simulink model "testEMplanner_cs"  (R2020b)
settings: Solver=FixedStepAuto  StartTime=0.0  StopTime=inf  FixedStep=1/1000  RelTol=1e-3
PreLoadFcn:
  | mbxruntime.callbacks.PreLoadFcn(bdroot);
PostLoadFcn:
  | mbxruntime.callbacks.PostLoadFcn(bdroot);
InitFcn:
  | mbxruntime.callbacks.InitFcn(bdroot);
StartFcn:
  | mbxruntime.callbacks.StartFcn(bdroot);
StopFcn:
  | mbxruntime.callbacks.StopFcn(bdroot);
model workspace: external: MAT-File testEMplanner_cs_hws.mat (data not in the file)
undefined symbols (not defined in the file): aubr, c_factor, cf, cr, DiscIntNeverNeededParam, global_path_x, global_path_y, KD_PID_distance, KD_PID_speed, KI_PID_distance, KI_PID_speed, KP_PID_distance, KP_PID_speed, la, lb, LQR_K1, LQR_K2, LQR_K3, LQR_K4, m, rack_displacement, right_wheel_ground, tablebr, vubr, vx_break_point
libraries: PreScanSimulinkLibrary x38, Solver_SF x1
(part 12 of 16)

== matlab function testEMplanner_cs/Audi_A8_Sedan_1/decision&planning module with quad1/EM Planner/obs/MATLAB Function2 ==
  data: x_set input; match_point_index_set output; y_set input; frenet_path_x input; frenet_path_y input; frenet_path_heading input; frenet_path_kappa input; proj_x_set output; proj_y_set output; proj_heading_set output; proj_kappa_set output
function [match_point_index_set,proj_x_set, proj_y_set,proj_heading_set,proj_kappa_set] = ...
    fcn(x_set,y_set,frenet_path_x,frenet_path_y,frenet_path_heading,frenet_path_kappa)
%该函数将批量计算x_set，y_set中的xy，在frenet_path下的投影的信息
%输入 x_set,y_set，待投影的点的集合
%x_set,y_set,frenet_path_x,frenet_path_y,frenet_path_heading,frenet_path_kappa
%曲线在直角坐标系下的x，y，heading，kappa
%输出：match_point_index_set 匹配点在frenet_path下的编号的集合(即从全局路径第一个点开始数，第几个点是匹配点)
%     proj_x y heading kappa 投影的x,y,heading,kappa的集合

% 由于事先不知道x_set中到底有多少个点需要投影，因此事先声明一个最大的数量的点作为缓冲
n = 128;
% 并且由于不知道投影点的个数，所以也不知道输出的个数，因此输出也要做缓冲，用nan表示不存在的点
% 输出最多输出128个
% 输出初始化
match_point_index_set = ones(n,1) * nan;
proj_x_set = ones(n,1) * nan;
proj_y_set = ones(n,1) * nan;
proj_heading_set = ones(n,1) * nan;
proj_kappa_set = ones(n,1) * nan;

% 找匹配点，需要利用上一个周期的结果作为下一个周期遍历的起点，因此需要声明两个全局变量

persistent is_first_run;
persistent pre_match_point_index_set;%bug :pre_match_point_index(i) 未必代表的是第i个障碍物的match_point_index
persistent pre_frenet_path_x;
persistent pre_frenet_path_y;
persistent pre_frenet_path_heading;
persistent pre_frenet_path_kappa;
persistent pre_x_set;
persistent pre_y_set;
%算法主函数入口

if isempty(is_first_run)
    %该if分支表示函数首次运行
    is_first_run = 0;
    pre_frenet_path_x = frenet_path_x;
    pre_frenet_path_y = frenet_path_y;
    pre_frenet_path_heading = frenet_path_heading;
    pre_frenet_path_kappa = frenet_path_kappa;
    %要记录首次运行计算的匹配点的结果供下个周期运行，先初始化
    pre_match_point_index_set = ones(n,1) * nan;
    %对x_set,y_set的点做遍历，找到他们的匹配点
    for i = 1 : length(x_set)
        if isnan(x_set(i))
            break;
        end
        %首次运行时，没有任何提示，只能从frenet path的第一个点开始找
        start_search_index = 1;
        % 声明increase_count，用于表示在遍历时distance连续增加的个数
        increase_count = 0;
        % 开始遍历
        min_distance = inf;
        for j = start_search_index : length(frenet_path_x)
            distance = (x_set(i) - frenet_path_x(j))^2 + (y_set(i) - frenet_path_y(j))^2;
            if distance < min_distance
                min_distance = distance;
                match_point_index_set(i) = j;
                increase_count = 0;
            else
                increase_count = increase_count + 1;
            end
            %如果distance连续增加50次就不要再遍历了，节省时间
            if increase_count > 50
                break;
            end
        end
        
        %如何通过匹配点计算投影点，请参见《自动驾驶控制算法第七讲》
        %或《自动驾驶决策规划算法》第一章第三节
        
        %取出匹配点的编号
        match_point_index = match_point_index_set(i);
        %取出匹配点的信息
        match_point_x = frenet_path_x(match_point_index);
        match_point_y = frenet_path_y(match_point_index);
        match_point_heading = frenet_path_heading(match_point_index);
        match_point_kappa = frenet_path_kappa(match_point_index);
        %计算匹配点的方向向量与法向量
        vector_match_point = [match_point_x;match_point_y];
        vector_match_point_direction = [cos(match_point_heading);sin(match_point_heading)];
        %声明待投影点的位矢
        vector_r = [x_set(i);y_set(i)];
        
       %通过匹配点计算投影点
       vector_d = vector_r - vector_match_point;
       ds = vector_d' * vector_match_point_direction;
       vector_proj_point = vector_match_point + ds * vector_match_point_direction;
       proj_heading = match_point_heading + match_point_kappa * ds;
       proj_kappa = match_point_kappa;
       %计算结果输出
       proj_x_set(i) = vector_proj_point(1);
       proj_y_set(i) = vector_proj_point(2);
       proj_heading_set(i) = proj_heading;
       proj_kappa_set(i) = proj_kappa;
    end
    %匹配点的计算结果保存，供下一个周期使用
    pre_match_point_index_set = match_point_index_set;
    pre_x_set = x_set;
    pre_y_set = y_set;
else
    %此if分支表示不是首次运行
    %对每个x_set上的点做处理
    for i = 1 : length(x_set)
        %不是首次运行，对于点x_set(i),y_set(i)来说,start_search_index =
        %pre_match_point_index_set(i)
        start_search_index = pre_match_point_index_set(i);%上个周期匹配点的编号作为本周期搜索的起点
        % 判断帧与帧之间的障碍物是否为同一个
        square_dis = (x_set(i) - pre_x_set(i))^2 + (y_set(i) - pre_y_set(i))^2;
        if square_dis > 36
            % 帧与帧之间的物体的位置距离过大，认为是两个障碍物
            start_search_index = nan;
        end
        % 声明increase_count，用于表示在遍历时distance连续增加的个数
        %%%%%%%%%
        %对于障碍物检测而言，当感知第一次检测到障碍物时，算法并不是首次运行，此时 
        %pre_match_point_index_set的值是nan，如果还用上一时刻的结果作为本周期搜索的起点
        %必然会出问题，所以要修改
        % 声明increase_count_limit
        increase_count_limit = 5;
        if isnan(start_search_index)
            %没有上个周期的结果，那就不能只检查5次了
            increase_count_limit = 50;
            %搜索起点也要设为1
            start_search_index = 1;
        end
        increase_count = 0;
        % 开始遍历
        %这里多一个步骤，判断遍历的方向
        %计算上个周期匹配点的位矢
        vector_pre_match_point = [pre_frenet_path_x(start_search_index);pre_frenet_path_y(start_search_index)];
        vector_pre_match_point_direction = ...
            [cos(pre_frenet_path_heading(start_search_index));sin(pre_frenet_path_heading(start_search_index))];
        %判断遍历的方向
        flag = ([x_set(i);y_set(i)] - vector_pre_match_point)' * vector_pre_match_point_direction;
        min_distance = inf;
        if flag > 0.001
            for j = start_search_index : length(frenet_path_x)
                distance = (x_set(i) - frenet_path_x(j))^2 + (y_set(i) - frenet_path_y(j))^2;
                if distance < min_distance
                    min_distance = distance;
                    match_point_index_set(i) = j;
                    increase_count = 0;
                else
                    increase_count = increase_count + 1;
                end
                %如果distance连续增加increase_count_limit次就不要再遍历了，节省时间
                if increase_count > increase_count_limit
                    break;
                end
            end
        elseif flag < - 0.001
            for j = start_search_index : -1 : 1
                distance = (x_set(i) - frenet_path_x(j))^2 + (y_set(i) - frenet_path_y(j))^2;
                if distance < min_distance
                    min_distance = distance;
                    match_point_index_set(i) = j;
                    increase_count = 0;
                else
                    increase_count = increase_count + 1;
                end
                %如果distance连续增加increase_count_limit次就不要再遍历了，节省时间
                if increase_count > increase_count_limit
                    break;
                end
            end
        else
            match_point_index_set(i) = start_search_index;
        end
        
        %如何通过匹配点计算投影点，请参见《自动驾驶控制算法第七讲》
        %或《自动驾驶决策规划算法》第一章第三节
        
        %取出匹配点的编号
        match_point_index = match_point_index_set(i);
        %取出匹配点的信息
        match_point_x = frenet_path_x(match_point_index);
        match_point_y = frenet_path_y(match_point_index);
        match_point_heading = frenet_path_heading(match_point_index);
        match_point_kappa = frenet_path_kappa(match_point_index);
        %计算匹配点的方向向量与法向量
        vector_match_point = [match_point_x;match_point_y];
        vector_match_point_direction = [cos(match_point_heading);sin(match_point_heading)];
        %声明待投影点的位矢
        vector_r = [x_set(i);y_set(i)];
        
       %通过匹配点计算投影点
       vector_d = vector_r - vector_match_point;
       ds = vector_d' * vector_match_point_direction;
       vector_proj_point = vector_match_point + ds * vector_match_point_direction;
       proj_heading = match_point_heading + match_point_kappa * ds;
       proj_kappa = match_point_kappa;
       %计算结果输出
       proj_x_set(i) = vector_proj_point(1);
       proj_y_set(i) = vector_proj_point(2);
       proj_heading_set(i) = proj_heading;
       proj_kappa_set(i) = proj_kappa;
  
    end
    %匹配点的计算结果保存，供下一个周期使用
    pre_match_point_index_set = match_point_index_set;
    pre_frenet_path_x = frenet_path_x;
    pre_frenet_path_y = frenet_path_y;
    pre_frenet_path_heading = frenet_path_heading;
    pre_frenet_path_kappa = frenet_path_kappa;
    pre_x_set = x_set;
    pre_y_set = y_set;
end

== matlab function testEMplanner_cs/Audi_A8_Sedan_1/decision&planning module with quad1/EM Planner/obs/obs filter ==
  data: host_x input; obs_x_set_final output; host_y input; host_heading_xy input; obs_x_set_gcs input; obs_y_set_gcs input; obs_velocity_set_gcs input; obs_heading_set_gcs input; obs_y_set_final output; obs_velocity_set_final output; obs_heading_set_final output
function [obs_x_set_final,obs_y_set_final,obs_velocity_set_final,obs_heading_set_final] = fcn(host_x,host_y,host_heading_xy,obs_x_set_gcs,obs_y_set_gcs,obs_velocity_set_gcs,obs_heading_set_gcs)
% 该函数将筛选障碍物，纵向[-10,60] 横向[-10,10]的障碍物才会被考虑
% 该函数只是一种单车道的临时办法，考虑到多车道情况，即使障碍物距离较远也应该考虑
% EM Planner完全体是多车道并行计算的，每个车道都生成参考线然后并行计算出多条轨迹，再选择最优的轨迹作为输出

%传感器最多可以识别32个障碍物
n = 32;
%输出初始化
obs_x_set_final = ones(n,1)*nan;
obs_y_set_final = ones(n,1)*nan;
obs_velocity_set_final = ones(n,1)*nan;
obs_heading_set_final = ones(n,1)*nan;
count = 1;
for i = 1:length(obs_x_set_gcs)
    if isnan(obs_x_set_gcs(i))
        break;
    end
    %自车的heading的方向向量与法向量
    tor = [cos(host_heading_xy);sin(host_heading_xy)];
    nor = [-sin(host_heading_xy);cos(host_heading_xy)];
    %障碍物与自车的距离向量
    vector_obs = [obs_x_set_gcs(i);obs_y_set_gcs(i)] - [host_x;host_y];
    %障碍物纵向距离
    lon_distance = vector_obs'*tor;
    %障碍物横向距离
    lat_distance = vector_obs'*nor;
    
    if (lon_distance < 60) && (lon_distance > -10) && (lat_distance > -10) && (lat_distance < 10)
        obs_x_set_final(count) = obs_x_set_gcs(i);
        obs_y_set_final(count) = obs_y_set_gcs(i);
        obs_heading_set_final(count) = obs_heading_set_gcs(i);
        obs_velocity_set_final(count) = obs_velocity_set_gcs(i);
        count = count + 1;
    end
end

== matlab function testEMplanner_cs/Audi_A8_Sedan_1/decision&planning module with quad1/EM Planner/path and speed merge ==
  data: s input; trajectory_x output; s_dot input; s_dot2 input; relative_time input; current_time input; path_s input; trajectory_x_init input; trajectory_y_init input; trajectory_heading_init input; trajectory_kappa_init input; trajectory_y output; trajectory_heading output; trajectory_kappa output; trajectory_speed output; trajectory_accel output; trajectory_time output
function [trajectory_x,trajectory_y,trajectory_heading,trajectory_kappa,trajectory_speed,trajectory_accel,trajectory_time] = ...
    fcn(s,s_dot,s_dot2,relative_time,current_time,path_s,trajectory_x_init,trajectory_y_init,trajectory_heading_init,trajectory_kappa_init)
% 该函数将合并path和speed
% 由于path 是 60个点，speed 有 401个点，合并后，path和speed有401个点，因此需要做插值
n = 401;
trajectory_x = zeros(n,1);
trajectory_y = zeros(n,1);
trajectory_heading = zeros(n,1);
trajectory_kappa = zeros(n,1);
trajectory_speed = zeros(n,1);

trajectory_accel = zeros(n,1);
index = 1;
% 由于trajectory_x_init中不是所有的值都有效，(有nan) 所以要找到有效值的范围
while ~isnan(trajectory_x_init(index)) 
    index = index + 1;
end
index = index - 1;
trajectory_time = zeros(n,1);
for i = 1:n-1
    %interp1 线性插值
    % 若 x = [1,2] y = [3,4]
    %interp1(x,y,1.5) 会得到3.5
    %interp1 的缺点是 在端点或超过端点的，结果为nan
    % interp1(x,y,2) 不会等于4 而是会等于nan
    % interp1(x,y,6) 也会等于nan，所以在端点处要单独处理
    trajectory_x(i) = interp1(path_s(1:index),trajectory_x_init(1:index),s(i));
    trajectory_y(i) = interp1(path_s(1:index),trajectory_y_init(1:index),s(i));
    trajectory_heading(i) = interp1(path_s(1:index),trajectory_heading_init(1:index),s(i));
    trajectory_kappa(i) = interp1(path_s(1:index),trajectory_kappa_init(1:index),s(i));
    trajectory_time(i) = relative_time(i) + current_time;%速度规划会得到相对时间，转换成绝对时间
    trajectory_speed(i) = s_dot(i);
    trajectory_accel(i) = s_dot2(i);
end
% 端点单独处理
trajectory_x(end) = trajectory_x_init(end);
trajectory_y(end) = trajectory_y_init(end);
trajectory_heading(end) = trajectory_heading_init(end);
trajectory_kappa(end) = trajectory_kappa_init(end);
trajectory_time(end) = relative_time(end) + current_time;
trajectory_speed(end) = s_dot(end);
trajectory_accel(end) = s_dot2(end);

== matlab function testEMplanner_cs/Audi_A8_Sedan_1/decision&planning module with quad1/EM Planner/path decision task/increase DP path nodes ==
  data: dp_path_s_init input; dp_path_s_final output; dp_path_l_init input; plan_start_s input; plan_start_l input; plan_start_dl input; plan_start_ddl input; dp_path_l_final output; dp_path_dl_final output; dp_path_ddl_final output
function [dp_path_s_final,dp_path_l_final,dp_path_dl_final,dp_path_ddl_final] = ...
    fcn(dp_path_s_init,dp_path_l_init,plan_start_s,plan_start_l,plan_start_dl,plan_start_ddl)
% 该函数将增密dp_path_s,dp_path_l
% 由于事先不知道动态规划采样的行和列，也就不知道动态规划计算的曲线有多长，因此需要做缓冲
% 每1“米”采样一个点，一共采60个
ds = 1;
% 输出初始化
dp_path_s_final = ones(60,1)*nan;
dp_path_l_final = ones(60,1)*nan;
dp_path_dl_final = ones(60,1)*nan;
dp_path_ddl_final = ones(60,1)*nan;

% 设置五次多项式的起点
start_s = plan_start_s;
start_l = plan_start_l;
start_dl = plan_start_dl;
start_ddl = plan_start_ddl;

s_cur = [];
l_temp = [];
dl_temp =[];
ddl_temp = [];

for i = 1:length(dp_path_s_init)
    if dp_path_s_init(i) == -1
        break;
    end
    for j = 1:10000
        %采样s
        s_node = start_s + ds*(j - 1);
        if s_node < dp_path_s_init(i)
            s_cur = [s_cur,s_node];
        else
            break;
        end
    end
    end_s = dp_path_s_init(i);
    end_l = dp_path_l_init(i);
    end_dl = 0;
    end_ddl = 0;
    coeff = CalcQuinticCoeffient(start_l,start_dl,start_ddl,end_l,end_dl,end_ddl,start_s,end_s);
    a0 = coeff(1);
    a1 = coeff(2);
    a2 = coeff(3);
    a3 = coeff(4);
    a4 = coeff(5);
    a5 = coeff(6);
    l = a0 * ones(1,length(s_cur)) + a1 * s_cur + a2 * s_cur.^2 + a3 * s_cur.^3 +...
        a4 * s_cur.^4 + a5 * s_cur.^5;
    dl = a1 * ones(1,length(s_cur)) + 2 * a2 * s_cur + 3 * a3 * s_cur.^2 + ...
        4 * a4 * s_cur.^3 + 5 * a5 * s_cur.^4;
    ddl = 2 * a2 * ones(1,length(s_cur)) + 6 * a3 * s_cur + 12 * a4 * s_cur.^2 + ...
        20 * a5 * s_cur.^3;
    % 把 l dl ddl 的结果保存
    l_temp = [l_temp,l];
    dl_temp = [dl_temp,dl];
    ddl_temp = [ddl_temp,ddl];
    % end的值赋值给start 做下一步循环
    start_s = end_s;
    start_l = end_l;
    start_dl = end_dl;
    start_ddl = end_ddl;
    s_cur = [];
end
   for k = 1:length(l_temp)
       if k == 61
           break;
       end
       dp_path_s_final(k) = plan_start_s + ds * (k - 1);
       dp_path_l_final(k) = l_temp(k);
       dp_path_dl_final(k) = dl_temp(k);
       dp_path_ddl_final(k) = ddl_temp(k);
   end
end

function coeff = CalcQuinticCoeffient(start_l,start_dl,start_ddl,end_l,end_dl,end_ddl,start_s,end_s)
    % l = a0 + a1*s + a2*s^2 + a3*s^3 + a4*s^4 + a5*s^5
    % l' = a1 + 2 * a2 * s + 3 * a3 * s^2 + 4 * a4 * s^3 + 5 * a5 * s^4
    % l'' = 2 * a2 + 6 * a3 * s + 12 * a4 * s^2 + 20 * a5 * s^3
    start_s2 = start_s * start_s;
    start_s3 = start_s2 * start_s;
    start_s4 = start_s3 * start_s;
    start_s5 = start_s4 * start_s;
    end_s2 = end_s * end_s;
    end_s3 = end_s2 * end_s;
    end_s4 = end_s3 * end_s;
    end_s5 = end_s4 * end_s;
    A = [1,start_s, start_s2,     start_s3,     start_s4,      start_s5;
         0 1,       2 * start_s,  3 * start_s2, 4 * start_s3,  5 * start_s4;
         0 0,       2,            6 * start_s,  12 * start_s2, 20 * start_s3;
         1,end_s, end_s2,     end_s3,     end_s4,      end_s5;
         0,1,     2 * end_s,  3 * end_s2, 4 * end_s3,  5 * end_s4;
         0,0,     2,          6 * end_s,  12 * end_s2, 20 * end_s3;];
    B = [start_l;
         start_dl;
         start_ddl;
         end_l;
         end_dl;
         end_ddl;];
     coeff = A \ B;
    
end

== matlab function testEMplanner_cs/Audi_A8_Sedan_1/decision&planning module V0.1/EM Planner/calc plan start info and stitch trajectory ==
  data: pre_trajectory_x input; plan_start_x output; pre_trajectory_y input; pre_trajectory_heading input; pre_trajectory_kappa input; pre_trajectory_velocity input; pre_trajectory_accel input; pre_trajectory_time input; current_time input; host_x input; host_y input; host_heading_xy input; host_vx input; host_vy input; host_ax input; host_ay input; plan_start_y output; plan_start_heading output; plan_start_kappa output; plan_start_vx output; plan_start_vy output; plan_start_ax output; plan_start_ay output; plan_start_time output; stitch_x output; stitch_y output; stitch_heading output; stitch_kappa output; stitch_speed output; stitch_accel output; stitch_time output
function [plan_start_x,plan_start_y,plan_start_heading,plan_start_kappa,plan_start_vx,plan_start_vy,plan_start_ax,...
    plan_start_ay,plan_start_time,stitch_x,stitch_y,stitch_heading,stitch_kappa,stitch_speed,stitch_accel,stitch_time] ...
    = fcn(pre_trajectory_x,pre_trajectory_y,pre_trajectory_heading,pre_trajectory_kappa,pre_trajectory_velocity,...
    pre_trajectory_accel,pre_trajectory_time,current_time,host_x,host_y,host_heading_xy,host_vx,host_vy,host_ax,host_ay)
%该函数将计算规划的起点以及拼接轨迹的信息
%输入 上一周期的规划结果信息pre_trajectory x ,y,heading,kappa,velocity,accel,time
%     本周期的绝对时间current_time
%     定位信息host x,y,heading,kappa,vx,vy,ax,ay
%输出 规划起点信息plan_start x,y,heading,kappa,vx,vy,ax,ay(vx,vy,ax,ay)是世界坐标系的
%     待拼接的轨迹信息，一般在上一周期的轨迹中的current_time+100ms，往前取20个点。
%     当规划完成后，本周期的规划结果和stitch_trajectory一起拼好发给控制

%输出初始化
stitch_x = zeros(20,1);
stitch_y = zeros(20,1);
stitch_heading = zeros(20,1);
stitch_kappa = zeros(20,1);
stitch_speed = zeros(20,1);
stitch_accel = zeros(20,1);
%时间为负代表没有对应的拼接轨迹
stitch_time = ones(20,1)*-1;

%申明全局变量
persistent is_first_run;
if isempty(is_first_run)
    %代表代码首次运行
    is_first_run = 0;
    %按照轨迹拼接算法，应该用车辆动力学递推，但是首次运行车辆的速度都是0，所以没必要递推了
    plan_start_x = host_x;
    plan_start_y = host_y;
    plan_start_heading = host_heading_xy;
    plan_start_kappa = 0;
    plan_start_vx = 0;
    plan_start_vy = 0;
    plan_start_ax = 0;
    plan_start_ay = 0;
    %规划的起点的时间应该是当前时间+100ms
    plan_start_time = current_time + 0.1;
else
    %该函数不是首次运行
    x_cur = host_x;
    y_cur = host_y;
    heading_cur = host_heading_xy;
    kappa_cur = 0;
    %vx vy ax ay要转换成世界坐标系
    vx_cur = host_vx*cos(heading_cur) - host_vy*sin(heading_cur);
    vy_cur = host_vx*sin(heading_cur) + host_vy*cos(heading_cur);
    ax_cur = host_ax*cos(heading_cur) - host_ay*sin(heading_cur);
    ay_cur = host_ax*sin(heading_cur) + host_ay*cos(heading_cur);
    %规划周期
    dt = 0.1;
    %由于不是首次运行了，有上一时刻的轨迹了，找到上一周期轨迹规划的本周期车辆应该在的位置
    for i = 1:length(pre_trajectory_time) - 1
        if (pre_trajectory_time(i) <= current_time && pre_trajectory_time(i + 1) > current_time)
            break;
        end
    end
    %上一周期规划的本周期的车应该在的位置
    pre_x_desire = pre_trajectory_x(i);
    pre_y_desire = pre_trajectory_y(i);
    pre_heading_desire = pre_trajectory_heading(i);
    %计算横纵向误差
    %切向量
    tor = [cos(pre_heading_desire);sin(pre_heading_desire)];
    %法向量
    nor = [-sin(pre_heading_desire);cos(pre_heading_desire)];
    %误差向量
    d_err = [host_x;host_y] - [pre_x_desire;pre_y_desire];
    %纵向误差
    lon_err = abs(d_err'*tor);
    %横向误差
    lat_err = abs(d_err'*nor);
    %纵向误差大于2.5 横向误差大于0.5 认为控制没跟上
    if (lon_err > 2.5)||(lat_err > 0.5)
        %此分支处理控制未跟上的情况，规划起点通过运动学递推
        plan_start_x = x_cur + vx_cur * dt + 0.5 * ax_cur * dt * dt;
        plan_start_y = y_cur + vy_cur * dt + 0.5 * ay_cur * dt * dt;
        plan_start_vx = vx_cur + ax_cur * dt;
        plan_start_vy = vy_cur + ay_cur * dt;
        plan_start_heading = atan2(plan_start_vy,plan_start_vx);
        plan_start_ax = ax_cur;
        plan_start_ay = ay_cur;
        plan_start_kappa = kappa_cur;
        plan_start_time = current_time + 0.1;
        return;
    else
        %此分支表示控制能跟的上规划，开始拼接
        for j = i:length(pre_trajectory_time) - 1
            if (pre_trajectory_time(j) <= current_time + 0.1)&&(pre_trajectory_time(j + 1) > current_time + 0.1)
                break;
            end
        end
        %注：此算法要能运行需要trajectory的点有很高的密度
        plan_start_x = pre_trajectory_x(j);
        plan_start_y = pre_trajectory_y(j);
        plan_start_heading = pre_trajectory_heading(j);
        plan_start_kappa = pre_trajectory_kappa(j);
        %这里的pre_trajectory的速度,加速度是指轨迹的切向速度，切向加速度
        plan_start_vx = pre_trajectory_velocity(j) * cos(plan_start_heading);
        plan_start_vy = pre_trajectory_velocity(j) * sin(plan_start_heading);
        %pre_trajectory的加速度是切向加速度，要想计算ax,ay还要计算法向加速度
        %计算轨迹在current_time + 100ms 这个点的切向量法向量
        tor = [cos(plan_start_heading);sin(plan_start_heading)];
        nor = [-sin(plan_start_heading);cos(plan_start_heading)];
        a_tor = pre_trajectory_accel(j) * tor;
        a_nor = pre_trajectory_velocity(j)^2 * plan_start_kappa * nor ;
        plan_start_ax = a_tor(1) + a_nor(1);
        plan_start_ay = a_tor(2) + a_nor(2);
        plan_start_time = pre_trajectory_time(j);
        %计算拼接轨迹
        %j 表示 current_time + 0.1 的时间点在 pre_trajectory_time的编号
        %拼接是往从j开始，往前拼接20个，也就是pre_trajectory(j-1),j-2,j-3,....j-19
        %分两种情况，如果j小于20，意味着前面的轨迹点不够20个
        %如果j >= 20,意味着前面的点多于20个
        %还有一个细节需要考虑，pre_trajectory x(j) y(j) ....是规划的起点，那么在轨迹拼接时
        %需不需要在stitch_trajectory中把pre_trajectory x(j) y(j) ....包含进去
        %答案是否定的，不应该包进去，因为规划的起点会在规划模块计算完成后的结果中包含，如果在拼接的时候
        %还要包含，那就等于规划起点包含了两次
        %除非本周期计算的轨迹不包含规划起点，那么stitch_trajectory可以包含规划起点。
        %如果本周期计算的轨迹包含规划起点，那么stitch_trajectory就不可以包含规划起点。
        %我们选择规划包含起点，拼接不包含起点的做法
        
        %把起点去掉
        j = j - 1;
        if j >= 20
            stitch_x = pre_trajectory_x(j - 19:j);
            stitch_y = pre_trajectory_y(j - 19:j);
            stitch_heading = pre_trajectory_heading(j - 19:j);
            stitch_kappa = pre_trajectory_kappa(j - 19:j);
            stitch_speed = pre_trajectory_velocity(j - 19:j);
            stitch_accel = pre_trajectory_accel(j - 19:j);
            stitch_time = pre_trajectory_time(j - 19:j);
        else
            stitch_x(20 - j + 1:20) = pre_trajectory_x(1:j);
            stitch_y(20 - j + 1:20) = pre_trajectory_y(1:j);
            stitch_heading(20 - j + 1:20) = pre_trajectory_heading(1:j);
            stitch_kappa(20 - j + 1:20) = pre_trajectory_kappa(1:j);
            stitch_speed(20 - j + 1:20) = pre_trajectory_velocity(1:j);
            stitch_accel(20 - j + 1:20) = pre_trajectory_accel(1:j);
            stitch_time(20 - j + 1:20) = pre_trajectory_time(1:j);           
        end   
    end    
end

== matlab function testEMplanner_cs/Audi_A8_Sedan_1/decision&planning module with quad1/EM Planner/path decision task/path decision with dynamic planning(dp) ==
  data: obs_s_set input; dp_path_s output; obs_l_set input; plan_start_s input; plan_start_l input; plan_start_dl input; plan_start_dll input; w_cost_collision input; w_cost_smooth_dl input; w_cost_smooth_ddl input; w_cost_smooth_dddl input; w_cost_ref input; row input; col input; sample_s input; sample_l input; dp_path_l output
function [dp_path_s,dp_path_l] = fcn(obs_s_set,obs_l_set,plan_start_s,plan_start_l,plan_start_dl,...
    plan_start_dll,w_cost_collision,w_cost_smooth_dl,w_cost_smooth_ddl,w_cost_smooth_dddl,w_cost_ref,row,col,sample_s,sample_l)
%该函数为路径决策算法动态规划的主函数
% 输入：obs s l set 筛选后的障碍物sl信息
%       plan_start s l dl ddl 规划起点信息
%       w_cost_obs,w_cost_smooth_dl,w_cost_smooth_ddl,w_cost_smooth_dddl,w_cost_ref动态规划代价权重
%       row col 动态规划采样点的行数和列数(row必须是奇数，col必须是6)
%       sample_s,sample_l 采样的s l 长度
% 输出：dp_path_l,dp_path_s 动态规划的路径sl,此路径不包含规划起点  

%动态规划最优的数据结构是结构体矩阵，但是simulink不支持结构体矩阵，所以动态规划算法写的相对难以理解

%声明二维矩阵变量node_cost，node_cost(i,j)表示从起点出发，到行i列j节点的最小代价为node_cost(i,j)
node_cost = ones(row,col)*inf;%初始化为无穷大

%声明二维矩阵变量pre_node_index pre_node_index(i,j)表示从起点到行i列j的节点的最优路径中前一个节点的行号为
%pre_node_index(i,j)
%例：比如一条最优路径为 起点 -> node(1,1) -> node(2,2) -> node(3,3)
%则pre_node_index(3,3) = 2 (最优路径的前一个节点是node(2,2) 取它的行号）
%  pre_node_index(2,2) = 1 (最优路径的前一个节点是node(1,1) 取它的行号）
%  pre_node_index(1,1) = 0 (起点的行号默认是0)

% 其实pre_node_index就是当找到最小代价的路径后从终点到起点反向选择出最优路径的
%如果用结构体矩阵完全没有必要弄得这么麻烦，但是simulink不支持
pre_node_index = zeros(row,col);%初始化，所有节点的上个最优节点的行号都是0，也就是起点

%先计算从起点到第一列的cost
for i = 1:row
    node_cost(i,1) = CalcStartCost(plan_start_s,plan_start_l,plan_start_dl,...
    plan_start_dll,i,sample_s,sample_l,w_cost_collision,w_cost_smooth_dl,...
    w_cost_smooth_ddl,w_cost_smooth_dddl,w_cost_ref,obs_s_set,obs_l_set,row);
end
% 动态规划主函数，从第二列开始
for j = 2:col
    for i = 1:row
        %计算当前node(i,j)的s l
        cur_node_s = plan_start_s + j * sample_s;
        cur_node_l = ((row + 1)/2 - i) * sample_l;
        %遍历前一列的节点
        for k = 1:row
            %计算前一列节点的s l
            pre_node_s = plan_start_s + (j - 1) * sample_s;
            pre_node_l = ((row + 1)/2 - k) * sample_l;
            cost_neighbour = CalcNeighbourCost(pre_node_s,pre_node_l,cur_node_s,cur_node_l,w_cost_collision,...
    w_cost_smooth_dl,w_cost_smooth_ddl,w_cost_smooth_dddl,w_cost_ref,obs_s_set,obs_l_set);
            %起点到上一个节点的最小代价为node_cost(k,j-1)
            pre_min_cost = node_cost(k,j-1);
            %起点到node_cost(i,j)的最小代价 为node_cost(k,j-1)
            %再加上node(k,j-1)到node(i,j)的代价 (k = 1,2,3,4...row) 中最小的
            cost_temp = pre_min_cost + cost_neighbour;
            if cost_temp < node_cost(i,j)
                node_cost(i,j) = cost_temp;
                %把最优路径上一列节点的行号记录下来
                pre_node_index(i,j) = k;
            end
        end      
    end
end
%找到node_cost最后一列中，cost最小的，记代价最小的行号为index
index = 0;
min_cost = inf;
for i = 1:row
    if node_cost(i,end) < min_cost
        min_cost = node_cost(i,end);
        index = i;
    end
end
%动态规划最优路径初始化
dp_node_list_row = zeros(col,1);
%从后往前逆推
cur_index = index;
for i = 1:col
    %记录cur_index前面节点的行号
    pre_index = pre_node_index(cur_index,end - i + 1);
    %把cur_index放到dp_node_list_row对应的位置
    dp_node_list_row(col - i + 1) = cur_index;
    %再把pre_index 赋给 cur_index 进行下一步递推
    cur_index = pre_index;
end
% 输出初始化，由于事先不知道横纵向的采样列数，因此需要做缓冲
dp_path_s = ones(15,1)*-1;
dp_path_l = ones(15,1)*-1;
for i = 1:col
    dp_path_s(i) = plan_start_s + i * sample_s;
    dp_path_l(i) = ((row + 1) / 2 - dp_node_list_row(i)) * sample_l;
end








end
function cost = CalcNeighbourCost(pre_node_s,pre_node_l,cur_node_s,cur_node_l,w_cost_collision,...
    w_cost_smooth_dl,w_cost_smooth_ddl,w_cost_smooth_dddl,w_cost_ref,obs_s_set,obs_l_set)
% 该函数将计算相邻两个节点之间的cost
  
    start_l = pre_node_l;
    start_dl = 0;
    start_ddl = 0;
    end_l = cur_node_l;
    end_dl = 0;
    end_ddl = 0;
    start_s = pre_node_s;
    end_s = cur_node_s;
    coeff = CalcQuinticCoeffient(start_l,start_dl,start_ddl,end_l,end_dl,end_ddl,start_s,end_s);
    a0 = coeff(1);
    a1 = coeff(2);
    a2 = coeff(3);
    a3 = coeff(4);
    a4 = coeff(5);
    a5 = coeff(6);
    % 取10个点计算cost
    ds = zeros(10,1);
    l = zeros(10,1);
    dl = zeros(10,1);
    ddl = zeros(10,1);
    dddl = zeros(10,1);
    for i = 1:10
        ds(i) = start_s + (i-1)*(end_s - start_s)/10;
    end
    l = a0 * ones(10,1) + a1 * ds + a2 * ds.^2 + a3 * ds.^3 + a4 * ds.^4 + a5 * ds.^5;
    dl = a1 * ones(10,1) + 2 * a2 * ds + 3 * a3 * ds.^2 + 4 * a4 * ds.^3 + 5 * a5 * ds.^4;
    ddl = 2 * a2 * ones(10,1) + 6 * a3 * ds + 12 * a4 * ds.^2 + 20 * a5 * ds.^3;
    dddl = 6 * ones(10,1) * a3 + 24 * a4 * ds + 60 * a5 * ds.^2;
    cost_smooth = w_cost_smooth_dl * (dl' * dl) + w_cost_smooth_ddl * (ddl' * ddl) + w_cost_smooth_dddl * (dddl' * dddl);
    for i = 1:length(ddl)
        if abs(ddl(i))> 0.5 || abs(atan(dl(i))) > 0.4*pi
            cost_smooth = cost_smooth + 1e7;
            break;
        end
    end
    cost_ref = w_cost_ref * (l' * l);
    cost_collision = 0;
    for i = 1:length(obs_s_set)
        if isnan(obs_s_set(i))
            break;
        end
        dlon = ones(10,1) * obs_s_set(i) - ds;
        dlat = ones(10,1) * obs_l_set(i) - l;
        %这里做了非常简化的质点模型，认为障碍物就是一个点
        square_d = dlon.^2 + dlat.^2;
        cost_collision_once = CalcObsCost(w_cost_collision,square_d);
        cost_collision = cost_collision + cost_collision_once;
        % 判断障碍物的左右
        v1 = [ds(end);l(end)] - [ds(1);l(1)];
        v2 = [obs_s_set(i);obs_l_set(i)] - [ds(1);l(1)];
        flag = v1(1)*v2(2) - v1(2)*v2(1);
        if flag < 0 && cost_collision > 0
            cost_collision = cost_collision - 1000;
        end
    end
    
    cost = cost_collision + cost_smooth + cost_ref;


end


function cost = CalcStartCost(begin_s,begin_l,begin_dl,begin_ddl,cur_node_row,sample_s,sample_l,w_cost_collision,...
    w_cost_smooth_dl,w_cost_smooth_ddl,w_cost_smooth_dddl,w_cost_ref,obs_s_set,obs_l_set,row)
    %该函数将计算起点到第一层的cost
    start_l = begin_l;
    start_dl = begin_dl;
    start_ddl = begin_ddl;
    %  . . .
    %  . . . row = 3 中间的行号 = (row + 1) /2 = 2
    %  . . .
    end_l = ((row + 1)/2 - cur_node_row)*sample_l;
    end_dl = 0;
    end_ddl = 0;
    start_s = begin_s;
    end_s = begin_s + sample_s;
    coeff = CalcQuinticCoeffient(start_l,start_dl,start_ddl,end_l,end_dl,end_ddl,start_s,end_s);
    a0 = coeff(1);
    a1 = coeff(2);
    a2 = coeff(3);
    a3 = coeff(4);
    a4 = coeff(5);
    a5 = coeff(6);
    % 取10个点计算cost
    ds = zeros(10,1);
    l = zeros(10,1);
    dl = zeros(10,1);
    ddl = zeros(10,1);
    dddl = zeros(10,1);
    for i = 1:10
        ds(i) = start_s + (i-1)*sample_s/10;
    end
    l = a0 * ones(10,1) + a1 * ds + a2 * ds.^2 + a3 * ds.^3 + a4 * ds.^4 + a5 * ds.^5;
    dl = a1 * ones(10,1) + 2 * a2 * ds + 3 * a3 * ds.^2 + 4 * a4 * ds.^3 + 5 * a5 * ds.^4;
    ddl = 2 * a2 * ones(10,1) + 6 * a3 * ds + 12 * a4 * ds.^2 + 20 * a5 * ds.^3;
    dddl = 6 * ones(10,1) * a3 + 24 * a4 * ds + 60 * a5 * ds.^2;
    cost_smooth = w_cost_smooth_dl * (dl' * dl) + w_cost_smooth_ddl * (ddl' * ddl) + w_cost_smooth_dddl * (dddl' * dddl);
    for i = 1:length(dl)
        if abs(ddl(i))> 0.5 || abs(atan(dl(i))) > 0.4*pi
            cost_smooth = cost_smooth + 1e7;
            break;
        end
    end
    cost_ref = w_cost_ref * (l' * l);
    cost_collision = 0;
    for i = 1:length(obs_s_set)
        if isnan(obs_s_set(i))
            break;
        end
        dlon = ones(10,1) * obs_s_set(i) - ds;
        dlat = ones(10,1) * obs_l_set(i) - l;
        %这里做了非常简化的质点模型，认为障碍物就是一个点
        square_d = dlon.^2 + dlat.^2;
        cost_collision_once = CalcObsCost(w_cost_collision,square_d);
        cost_collision = cost_collision + cost_collision_once;
        % 判断障碍物的左右
        v1 = [ds(end);l(end)] - [ds(1);l(1)];
        v2 = [obs_s_set(i);obs_l_set(i)] - [ds(1);l(1)];
        flag = v1(1)*v2(2) - v1(2)*v2(1);
        if flag < 0 && cost_collision > 0
            cost_collision = cost_collision - 1000;
        end
    end
    
    cost = cost_collision + cost_smooth + cost_ref;
        
end

function obs_cost = CalcObsCost(w_cost_collision,square_d)
%该函数将计算障碍物的距离代价
% 暂定超过4米的cost为0 在4到3米的cost为1000/squard_d,在小于3米的cost为w_cost_collision
%   cost = 0;
%   for i = 1:length(square_d)
%       if (square_d(i) < 16 && square_d(i) > 9) 
%           cost = cost + 500/square_d(i);
%       elseif (square_d(i) <= 9)
%           cost = cost + w_cost_collision;
%       end
%   end
%   obs_cost = cost;
min_d = inf;
for i = 1:length(square_d)
    min_d = min(min_d,square_d(i));
end
    obs_cost = w_cost_collision * 10^(-min_d/3);
end

function coeff = CalcQuinticCoeffient(start_l,start_dl,start_ddl,end_l,end_dl,end_ddl,start_s,end_s)
    % l = a0 + a1*s + a2*s^2 + a3*s^3 + a4*s^4 + a5*s^5
    % l' = a1 + 2 * a2 * s + 3 * a3 * s^2 + 4 * a4 * s^3 + 5 * a5 * s^4
    % l'' = 2 * a2 + 6 * a3 * s + 12 * a4 * s^2 + 20 * a5 * s^3
    start_s2 = start_s * start_s;
    start_s3 = start_s2 * start_s;
    start_s4 = start_s3 * start_s;
    start_s5 = start_s4 * start_s;
    end_s2 = end_s * end_s;
    end_s3 = end_s2 * end_s;
    end_s4 = end_s3 * end_s;
    end_s5 = end_s4 * end_s;
    A = [1,start_s, start_s2,     start_s3,     start_s4,      start_s5;
         0 1,       2 * start_s,  3 * start_s2, 4 * start_s3,  5 * start_s4;
         0 0,       2,            6 * start_s,  12 * start_s2, 20 * start_s3;
         1,end_s, end_s2,     end_s3,     end_s4,      end_s5;
         0,1,     2 * end_s,  3 * end_s2, 4 * end_s3,  5 * end_s4;
         0,0,     2,          6 * end_s,  12 * end_s2, 20 * end_s3;];
    B = [start_l;
         start_dl;
         start_ddl;
         end_l;
         end_dl;
         end_ddl;];
     coeff = A \ B;
    
end

== matlab function testEMplanner_cs/Audi_A8_Sedan_1/decision&planning module with quad1/EM Planner/path planning task/generate convex space ==
  data: dp_path_s input; l_min output; dp_path_l input; static_obs_s_set input; static_obs_l_set input; static_obs_length input; static_obs_width input; l_max output
function [l_min,l_max] = fcn(dp_path_s,dp_path_l,static_obs_s_set,static_obs_l_set,static_obs_length,static_obs_width)
    % 该函数将输出每个离散的dp_path_s所对应的l的边界lmin lmax (本质上是质点的凸空间)
    % 输入 动态规划曲线 dp_path_s,dp_path_l
    %      障碍物中心的s l 坐标 static_obs_s,static_obs_l
    %      障碍物的长宽 static_obs_length,static_obs_width 
    % 输出 l_min lmax l 的上下界

    % 输出初始化
    l_min = ones(60,1) * -8;
    l_max = ones(60,1) * 8;
    % 对每个障碍物做遍历
    for i = 1:length(static_obs_s_set)
        if isnan(static_obs_s_set(i))
            break;
        end
        % 计算障碍物的头部和尾部的s
        obs_s_min = static_obs_s_set(i) - static_obs_length/2;
        obs_s_max = static_obs_s_set(i) + static_obs_length/2;
        % 找到dp_path_s 中，与s_head s_end最近的s的编号
        start_index = FindNearIndex(dp_path_s,obs_s_min);
        end_index = FindNearIndex(dp_path_s,obs_s_max);
        path_l = (dp_path_l(start_index) + dp_path_l(end_index))/2;
        if start_index == 1 && end_index == 1
            continue;
        end
        if path_l > static_obs_l_set(i)
            % 意味着决策为向左绕过障碍物
            for j = start_index:end_index
                % l_min(j) 为所有决策为向左绕过障碍物的l边界的最大值
                l_min(j) = max(l_min(j) , static_obs_l_set(i) + static_obs_width/2);
            end
        else
            % 意味着决策为向右绕过障碍物
            for j = start_index:end_index
                % l_max(j) 为所有决策为向右绕过障碍物的l边界的最小值
                l_max(j) = min(l_max(j) , static_obs_l_set(i) - static_obs_width/2);
            end
        end       
    end
end

function y = FindNearIndex(dp_path_s,obs_s)
    % 该函数将找到dp_path_s的所有点中，距离obs_s最近的点的编号
    % 这里要注意obs_s 是在完整的reference line上投影所得到的坐标，所以obs_s可能是负值，也可能会超过dp_path_s最远的长度
    if dp_path_s(1) >= obs_s
        %障碍物在后面
        y = 1;
        return;
    elseif dp_path_s(end) <= obs_s
        y = 60;
        return;
    else
        index = 1;
        while dp_path_s(index) < obs_s
            index = index + 1;
        end
        % 循环退出的条件是dp_path_s(index) >= obs_s 判断一下index 和 index-1哪个离的近
        if dp_path_s(index) - obs_s > obs_s - dp_path_s(index - 1)
            y = index - 1;
        else
            y = index;
        end
    end
end

== matlab function testEMplanner_cs/Audi_A8_Sedan_1/decision&planning module with quad1/EM Planner/path planning task/path planning with quadratic programming (qp) ==
  data: l_min input; qp_path_l output; l_max input; w_cost_l input; w_cost_dl input; w_cost_ddl input; w_cost_dddl input; w_cost_centre input; w_cost_end_l input; w_cost_end_dl input; w_cost_end_ddl input; host_d1 input; host_d2 input; host_w input; plan_start_l input; plan_start_dl input; plan_start_ddl input; qp_path_dl output; qp_path_ddl output; dp_path_l_final input
function [qp_path_l,qp_path_dl,qp_path_ddl] = ...
fcn(l_min,l_max,w_cost_l,w_cost_dl,w_cost_ddl,w_cost_dddl,w_cost_centre,w_cost_end_l,w_cost_end_dl,w_cost_end_ddl,...
    host_d1,host_d2,host_w,...
    plan_start_l,plan_start_dl,plan_start_ddl,dp_path_l_final)
% 路径二次规划
% 0.5*x'Hx + f'*x = min
% subject to A*x <= b
%            Aeq*x = beq
%            lb <= x <= ub;
% 输入：l_min l_max 点的凸空间
%       w_cost_l 参考线代价
%       w_cost_dl ddl dddl 光滑性代价
%       w_cost_centre 凸空间中央代价
%       w_cost_end_l dl dd1 终点的状态代价 (希望path的终点状态为(0,0,0))
%       host_d1,d2 host质心到前后轴的距离
%       host_w host的宽度
%       plan_start_l,dl,ddl 规划起点
% 输出 qp_path_l dl ddl 二次规划输出的曲线
coder.extrinsic("quadprog");
% 待优化的变量的数量
n = 60;

% 输出初始化
qp_path_l = zeros(n,1);
qp_path_dl = zeros(n,1);
qp_path_ddl = zeros(n,1);
% H_L H_DL H_DDL H_DDDL Aeq beq A b 初始化
H_L = zeros(3*n, 3*n);
H_DL = zeros(3*n, 3*n);
H_DDL = zeros(3*n, 3*n);
H_DDDL = zeros(n-1, 3*n);
H_CENTRE = zeros(3*n, 3*n);
H_L_END = zeros(3*n, 3*n);
H_DL_END = zeros(3*n, 3*n);
H_DDL_END = zeros(3*n, 3*n);
Aeq = zeros(2*n-2, 3*n);
beq = zeros(2*n-2, 1);
A = zeros(8*n, 3*n);
b = zeros(8*n, 1);
%  期望的终点状态
end_l_desire = 0;
end_dl_desire = 0;
end_ddl_desire = 0;

% Aeq_sub
ds = 1;%纵向间隔
Aeq_sub = [1 ds ds^2/3 -1 0 ds^2/6;
           0 1  ds/2   0 -1 ds/2];
% A_sub;
d1 = host_d1;
d2 = host_d2;
w = host_w;
A_sub = [1  d1 0;
         1  d1 0;
         1 -d2 0;
         1 -d2 0;
        -1 -d1 0;
        -1 -d1 0;
        -1  d2 0;
        -1  d2 0];
% 生成Aeq
for i = 1:n-1
    % 计算分块矩阵左上角的行和列
    row = 2*i - 1;
    col = 3*i - 2;
    Aeq(row:row + 1,col:col + 5) = Aeq_sub;
end
% 生成A
for i = 1:n
    row = 8*i - 7;
    col = 3*i - 2;
    A(row:row + 7,col:col + 2) = A_sub;
end

% 视频里用的找(s(i) - d2,s(i) + d1)的方法过于保守，在这里舍弃掉
% 只要找到四个角点所对应的l_min l_max 即可
% 。。。。。。。。。。。。。。
%    [    .   ]<- 
%    [        ]
% 。。。。。。。。。。。。。
front_index = ceil(d1/ds);
back_index = ceil(d2/ds); % ceil向上取整 ceil(3) = 3 ceil(3.1) = 4
% 生成b
for i = 1:n
    % 左前 右前的index = min(i + front_index,60)
    % 左后 右后的index = max(i - back_index,1)
    index1 = min(i + front_index,n);
    index2 = max(i - back_index,1);
    b(8*i - 7:8*i,1) = [l_max(index1) - w/2;
                        l_max(index1) + w/2;
                        l_max(index2) - w/2;
                        l_max(index2) + w/2;
                       -l_min(index1) + w/2;
                       -l_min(index1) - w/2;
                       -l_min(index2) + w/2;
                       -l_min(index2) - w/2;];
end
%生成 lb ub 主要是对规划起点做约束
lb = ones(3*n,1)*-inf;
ub = ones(3*n,1)*inf;
% lb(1) = - plan_start_l;
% lb(2) = -0.1;
% lb(3) = -0.1;
% ub(1) = plan_start_l;
% ub(2) = 0.1;
% ub(3) = 0.1;
lb(1) = plan_start_l;
lb(2) = plan_start_dl;
lb(3) = plan_start_ddl;
ub(1) = lb(1);
ub(2) = lb(2);
ub(3) = lb(3);
for i = 2:n
    lb(3*i - 1) = - pi/8;
    ub(3*i - 1) = pi/8;
    lb(3*i) = -0.1;
    ub(3*i) = 0.1;
end
% 生成H_L,H_DL,H_DDL,H_CENTRE
for i = 1:n
    H_L(3*i - 2,3*i - 2) = 1;
    H_DL(3*i - 1,3*i - 1) = 1;
    H_DDL(3*i, 3*i) = 1;
end
H_CENTRE = H_L;
% 生成H_DDDL;
H_dddl_sub = [0 0 1 0 0 -1];
for i = 1:n-1
    row = i;
    col = 3*i - 2;
    H_DDDL(row,col:col + 5) = H_dddl_sub;
end
% 生成H_L_END H_DL_END H_DDL_END
H_L_END(3*n - 2,3*n - 2) = 1;
H_DL_END(3*n - 1,3*n - 1) = 1;
H_DDL_END(3*n,3*n) = 1;
% 生成二次规划的H
H = w_cost_l * (H_L'*H_L) + w_cost_dl * (H_DL'*H_DL) + w_cost_ddl * (H_DDL'*H_DDL)...
   +w_cost_dddl * (H_DDDL'*H_DDDL) + w_cost_centre * (H_CENTRE'*H_CENTRE) + w_cost_end_l * (H_L_END'*H_L_END)...
   +w_cost_end_dl * (H_DL_END'* H_DL_END) + w_cost_ddl * (H_DDL_END'*H_DDL_END);
H = 2 * H;
% 生成f
f = zeros(3*n,1);
centre_line = 0.5 * (l_min + l_max);
centre_line = dp_path_l_final;
for i = 1:n
    f(3*i - 2) = -2 * centre_line(i);
end

f = w_cost_centre * f;
% 终点要接近end_l dl ddl desire
f(3*n - 2) = f(3*n - 2) -2 * end_l_desire * w_cost_end_l;
f(3*n - 1) = f(3*n - 1) -2 * end_dl_desire * w_cost_end_dl;
f(3*n) = f(3*n) -2 * end_ddl_desire * w_cost_end_ddl;

X0 = zeros(3*n,1);
%for i = 1 : n
X0(1) = plan_start_l;
X0(2) = plan_start_dl;
X0(3) = plan_start_ddl;

% X = quadprog(H,f,A,b,Aeq,beq,lb,ub,X0);
% X = quadprog(H,f,A,b);
X = quadprog(H,f,A,b,Aeq,beq);

% 这里没有对曲率做强制约束，并不好
% 可以用 |dl(i+1) - dl(i)|/ds <= kappa_max 近似去约束曲率
for i = 1:n
    qp_path_l(i) = X(3*i - 2);
    qp_path_dl(i) = X(3*i - 1);
    qp_path_ddl(i) = X(3*i);
end

end

== matlab function testEMplanner_cs/Audi_A8_Sedan_1/decision&planning module with quad1/EM Planner/plot ==
  data: dp_s input; dp_l input; qp_l input; l_min input; l_max input; obs_s_set input; obs_l_set input; start_s input; start_l input; start_dl input
function  fcn(dp_s,dp_l,qp_l,l_min,l_max,obs_s_set,obs_l_set,start_s,start_l,start_dl)
coder.extrinsic("plot","axis","figure","drawnow","cla","fill");

obs_length = 5;
obs_width = 2;
host_l = 6;
host_w = 1.63;
cla;
host_p1_l = start_l + sin(atan(start_dl)) * host_l /2 + host_w/2 * cos(atan(start_dl));
host_p1_s = start_s + cos(atan(start_dl)) * host_l /2 - host_w/2 * sin(atan(start_dl));
host_p2_l = start_l + sin(atan(start_dl)) * host_l /2 - host_w/2 * cos(atan(start_dl));
host_p2_s = start_s + cos(atan(start_dl)) * host_l /2 + host_w/2 * sin(atan(start_dl));
host_p3_l = start_l - sin(atan(start_dl)) * host_l /2 + host_w/2 * cos(atan(start_dl));
host_p3_s = start_s - cos(atan(start_dl)) * host_l /2 - host_w/2 * sin(atan(start_dl));
host_p4_l = start_l - sin(atan(start_dl)) * host_l /2 - host_w/2 * cos(atan(start_dl));
host_p4_s = start_s - cos(atan(start_dl)) * host_l /2 + host_w/2 * sin(atan(start_dl));
host_area_x = [host_p1_s;host_p2_s;host_p4_s;host_p3_s];
host_area_y = [host_p1_l;host_p2_l;host_p4_l;host_p3_l];
fill(host_area_x,host_area_y,[0 1 1]);
hold on
plot(dp_s,dp_l,'r');

plot(dp_s,qp_l,'b');
plot(dp_s,l_min,dp_s,l_max);
axis([-8 70 -10 10]);

for i = 1:length(obs_s_set)
    if isnan(obs_s_set(i))
        break;
    end
    obs_p1_s = obs_s_set(i) + obs_length/2;
    obs_p1_l = obs_l_set(i) + obs_width/2;
    obs_p2_s = obs_s_set(i) + obs_length/2;
    obs_p2_l = obs_l_set(i) - obs_width/2;
    obs_p3_s = obs_s_set(i) - obs_length/2;
    obs_p3_l = obs_l_set(i) + obs_width/2;
    obs_p4_s = obs_s_set(i) - obs_length/2;
    obs_p4_l = obs_l_set(i) - obs_width/2;
    obs_area_s = [obs_p1_s;obs_p2_s;obs_p4_s;obs_p3_s];
    obs_area_l = [obs_p1_l;obs_p2_l;obs_p4_l;obs_p3_l];
    fill(obs_area_s,obs_area_l,[0 0 0]);
end

== matlab function testEMplanner_cs/Audi_A8_Sedan_1/decision&planning module with quad1/EM Planner/simple speed qp planning ==
  data: plan_start_s_dot input; s_init output; plan_start_s_dot2 input; s_end input; recommend_T input; s_dot_init output; s_dot2_init output; relative_time_init output
function [s_init,s_dot_init,s_dot2_init,relative_time_init] = fcn(plan_start_s_dot,plan_start_s_dot2,s_end,recommend_T)
%简单速度二次规划
coder.extrinsic("quadprog")
n = 51;
s_init = zeros(n,1);
s_dot_init = zeros(n,1);
s_dot2_init = zeros(n,1);
relative_time_init = zeros(n,1);

Aeq = zeros(3*n,2*n - 2);
beq = zeros(2*n - 2,1);
lb = ones(3*n,1);
ub = lb;
dt = recommend_T/(n-1);
A_sub =[1,0;
        dt,1;
        (1/3)*dt^2,(1/2)*dt;
        -1,0;
        0,-1;
        (1/6)*dt^2,dt/2];
for i = 1:n - 1
    Aeq(3*i-2:3*i+3,2*i-1:2*i) = A_sub;
end

for i = 1:n
   lb(3*i - 2) = -inf;
   lb(3*i - 1) = 0;
   lb(3*i) = -8;
   ub(3*i - 2) = inf;
   ub(3*i - 1) = 50;
   ub(3*i) = 2;
end
lb(1) = 0;
lb(2) = plan_start_s_dot;
lb(3) = plan_start_s_dot2;
ub(1) = lb(1);
ub(2) = lb(2);
ub(3) = lb(3);
lb(3*n - 2) = s_end;
ub(3*n - 2) = s_end;
A3 = zeros(3*n,3*n);
A4 = zeros(3*n,n - 1);
A4_sub =[0;0;1;0;0;-1];
for i = 1:n - 1
   A3(3*i,3*i) = 1;
   A4(3*i-2:3*i+3,i:i) = A4_sub;
end
A3(3*n,3*n) = 1;
H = A3 + 100*(A4*A4');
H = 2*H;
f = zeros(3*n,1);
X = quadprog(H,f,[],[],Aeq',beq,lb,ub);
for i = 1:n
   s_init(i) = X(3*i - 2);
   s_dot_init(i) = X(3*i - 1);
   s_dot2_init(i) = X(3*i);
   relative_time_init(i) = (i - 1)*dt;
end

== matlab function testEMplanner_cs/Audi_A8_Sedan_1/decision&planning module with quad1/EM Planner/stitch trajectory ==
  data: trajectory_x input; trajectory_x_final output; trajectory_y input; trajectory_heading input; trajectory_kappa input; trajectory_speed input; trajectory_accel input; trajectory_time input; stitch_x input; stitch_y input; stitch_heading input; stitch_kappa input; stitch_speed input; stitch_accel input; stitch_time input; trajectory_y_final output; trajectory_heading_final output; trajectory_kappa_final output; trajectory_speed_final output; trajectory_accel_final output; trajectory_time_final output
function [trajectory_x_final,trajectory_y_final,trajectory_heading_final,trajectory_kappa_final,...
          trajectory_speed_final,trajectory_accel_final,trajectory_time_final] = fcn(trajectory_x,...
          trajectory_y,trajectory_heading,trajectory_kappa,trajectory_speed,trajectory_accel,trajectory_time,...
          stitch_x,stitch_y,stitch_heading,stitch_kappa,stitch_speed,stitch_accel,stitch_time)
% 轨迹拼接，把stitch trajectory 拼到规划完成的轨迹上
n = 401 + 20;
trajectory_x_final = zeros(n,1);
trajectory_y_final = zeros(n,1);
trajectory_heading_final = zeros(n,1);
trajectory_kappa_final = zeros(n,1);
trajectory_speed_final = zeros(n,1);
trajectory_accel_final = zeros(n,1);
trajectory_time_final = zeros(n,1);

trajectory_x_final = [stitch_x;trajectory_x];
trajectory_y_final = [stitch_y;trajectory_y];
trajectory_heading_final = [stitch_heading;trajectory_heading];
trajectory_kappa_final = [stitch_kappa;trajectory_kappa];
trajectory_speed_final = [stitch_speed;trajectory_speed];
trajectory_accel_final = [stitch_accel;trajectory_accel];
trajectory_time_final = [stitch_time;trajectory_time];

== matlab function testEMplanner_cs/Audi_A8_Sedan_1/decision&planning module with quad1/referenceline provider/MATLAB Function1 ==
  data: path_x input; path_heading output; path_y input; path_kappa output
function [path_heading,path_kappa] = fcn(path_x,path_y)
%该函数将计算path的切线方向与x轴的夹角和曲率
%输入：path_x,y路径坐标
%输出：path heading kappa 路径的heading和曲率
%原理 heading = arctan(dy/dx);
%     kappa = dheading/ds;
%     ds = (dx^2 + dy^2)^0.5

%注意，角度的多值性会带来很大的麻烦，需要慎重处理
%例，x 与 x + 2pi往往代表同一个角度，这种多值性在计算曲率会带来麻烦
%比如 原本是(0.1 - (-0.1))/ds，但如果计算出的-0.1多了一个2pi
%kappa就等于(0.1 - (-0.1 + 2*pi))/ds，曲率会变得非常大
%还有若采用中点欧拉法计算heading时，(即使用(y2 - y1)/(x2 - x1)的反正切计算一个角度 ，用(y1 - y0)/(x1
%-x0)的反正切又计算一个角度，然后加起来除以2),如果精确值是 (a1 + a2)/2,但最终计算的结果可能是(a1 + a2 + 2pi)/2
% 还有 tan(x) = tan(x + pi) 所以arctan(tan(x))可能等于x，也可能等于x + pi
% 角度的处理非常麻烦，而且角度处理不当往往是许多奇怪错误的源头

dx = diff(path_x);
dy = diff(path_y);
%用中点欧拉法要比向前欧拉法向后欧拉法更精确，但是也可能计算出的结果比精确值多一个pi
%在这里对dx,dy做中点欧拉法，使用四象限反正切计算角度
dx_pre = [dx(1);dx];
dx_after = [dx;dx(end)];
dx_final = (dx_pre + dx_after)/2;

dy_pre = [dy(1);dy];
dy_after = [dy;dy(end)];
dy_final = (dy_pre + dy_after)/2;

ds_final = sqrt(dx_final.^2 + dy_final.^2);
path_heading = atan2(dy_final,dx_final);

dheading = diff(path_heading);
dheading_pre = [dheading(1);dheading];
dheading_after = [dheading;dheading(end)];
dheading_final = (dheading_pre + dheading_after) / 2;
%为了防止dheading出现多一个2pi的错误，假设真实的dheading较小，用sin(dheading)近似dheading
path_kappa = sin(dheading_final) ./ ds_final;

== matlab function testEMplanner_cs/Audi_A8_Sedan_1/decision&planning module with quad1/referenceline provider/MATLAB Function2 ==
  data: host_match_point_index input; referenceline_x_init output; global_path_x input; global_path_y input; referenceline_y_init output
function [referenceline_x_init,referenceline_y_init] = fcn(host_match_point_index,global_path_x,global_path_y)
%该函数将在全局路径上提取referenceline的未平滑的初值
%输入： host_match_point_index 自车的位置在全局路径的匹配点的编号
       %global_path_x,global_path_y 全局路径数据
%输出：referenceline_x_init,referenceline_y_init 未平滑的参考线的xy坐标

%由于global path 是每1m取一个点，所以从匹配点往后取30个点，往前取150个点即可，一共181个点
%后面的点不够的话就用前面的点补，前面的点不够的话就用后面的点补，保证总数是181个

%索引初始化
start_index = -1;
%判断后面前面的点是否足够多
if host_match_point_index - 30 < 1
    %匹配点后面的点太少了，不够30个
    start_index = 1;
elseif host_match_point_index + 150 > length(global_path_x)
    %匹配点前面的点太少了，不够150个
    start_index = length(global_path_x) - 180;
    
else
    %匹配点正常情况
    start_index = host_match_point_index - 30;
end
%提取referenceline
referenceline_x_init = global_path_x(start_index:start_index + 180);
referenceline_y_init = global_path_y(start_index:start_index + 180);

== matlab function testEMplanner_cs/Audi_A8_Sedan_1/decision&planning module with quad1/referenceline provider/MATLAB Function3 ==
  data: path_x input; path_heading output; path_y input; path_kappa output
function [path_heading,path_kappa] = fcn(path_x,path_y)
%该函数将计算path的切线方向与x轴的夹角和曲率
%输入：path_x,y路径坐标
%输出：path heading kappa 路径的heading和曲率
%原理 heading = arctan(dy/dx);
%     kappa = dheading/ds;
%     ds = (dx^2 + dy^2)^0.5

%注意，角度的多值性会带来很大的麻烦，需要慎重处理
%例，x 与 x + 2pi往往代表同一个角度，这种多值性在计算曲率会带来麻烦
%比如 原本是(0.1 - (-0.1))/ds，但如果计算出的-0.1多了一个2pi
%kappa就等于(0.1 - (-0.1 + 2*pi))/ds，曲率会变得非常大
%还有若采用中点欧拉法计算heading时，(即使用(y2 - y1)/(x2 - x1)的反正切计算一个角度 ，用(y1 - y0)/(x1
%-x0)的反正切又计算一个角度，然后加起来除以2),如果精确值是 (a1 + a2)/2,但最终计算的结果可能是(a1 + a2 + 2pi)/2
% 还有 tan(x) = tan(x + pi) 所以arctan(tan(x))可能等于x，也可能等于x + pi
% 角度的处理非常麻烦，而且角度处理不当往往是许多奇怪错误的源头

dx = diff(path_x);
dy = diff(path_y);
%用中点欧拉法要比向前欧拉法向后欧拉法更精确，但是也可能计算出的结果比精确值多一个pi
%在这里对dx,dy做中点欧拉法，使用四象限反正切计算角度
dx_pre = [dx(1);dx];
dx_after = [dx;dx(end)];
dx_final = (dx_pre + dx_after)/2;

dy_pre = [dy(1);dy];
dy_after = [dy;dy(end)];
dy_final = (dy_pre + dy_after)/2;

ds_final = sqrt(dx_final.^2 + dy_final.^2);
path_heading = atan2(dy_final,dx_final);

dheading = diff(path_heading);
dheading_pre = [dheading(1);dheading];
dheading_after = [dheading;dheading(end)];
dheading_final = (dheading_pre + dheading_after) / 2;
%为了防止dheading出现多一个2pi的错误，假设真实的dheading较小，用sin(dheading)近似dheading
path_kappa = sin(dheading_final) ./ ds_final;
